simulink model "EV_Truck_Model"  (R2022b)
settings: Solver=FixedStepAuto  StartTime=0  StopTime=26553  FixedStep=0.1  RelTol=1e-3
model workspace (MAT data in the model file):
  ADAS_MaxAccel = 2
  ADAS_MaxDecel = 2.5
  Adas_on_off = 0
  Batt_cap_ah : Simulink.Parameter (value not decoded)
  Batt_rist_r0 : Simulink.Parameter (value not decoded)
  Batt_soc_s0 : Simulink.Parameter (value not decoded)
  Batt_volt_v0 : Simulink.Parameter (value not decoded)
  Motor_eff_100 : Simulink.Parameter (value not decoded)
  Motor_eff_190 : Simulink.Parameter (value not decoded)
  Motor_eff_95 : Simulink.Parameter (value not decoded)
  Motor_rpm_100 : Simulink.Parameter (value not decoded)
  Motor_rpm_190 : Simulink.Parameter (value not decoded)
  Motor_rpm_95 : Simulink.Parameter (value not decoded)
  Motor_torque_pos_100 : Simulink.Parameter (value not decoded)
  Motor_torque_pos_190 : Simulink.Parameter (value not decoded)
  Motor_torque_pos_95 : Simulink.Parameter (value not decoded)
  Motor_trq_190 : Simulink.Parameter (value not decoded)
  Motor_trq_95 : Simulink.Parameter (value not decoded)
  Sim_step = 0.1
  Test_DriveCycle = 0
  Trans_ratio = 6.142
  Veh_cog_fx = 1.69543
  Veh_cog_h = 0.605887
  Veh_cog_rx = 2.11956
  Veh_diff = 6.7
  Veh_whl_crr = 0.01
  Veh_whl_k = 180000
  Veh_whl_radius = 0.35
symbols that are objects in the model workspace (value not decoded): Motor_eff_100, Motor_eff_190, Motor_eff_95, Motor_rpm_100, Motor_rpm_190, Motor_rpm_95, Motor_torque_pos_100, Motor_torque_pos_190, Motor_torque_pos_95, Motor_trq_190, Motor_trq_95
undefined symbols (not defined in the file): Batt_soc_init, canChannel, Elec_aux_sw, Elec_rgn_sw, Power_option, speed, time, Veh_mass
libraries: batteryecm_lib x170, simulink x14, canmsglib x9, canlib x7, autolibshared x5, nesl_utility x4, fl_lib x3, drivingvehiclecontroller x3, hdlsllib x3, sim3dlib x1, sim3dautolib x1, vrlib x1
(part 4 of 11)

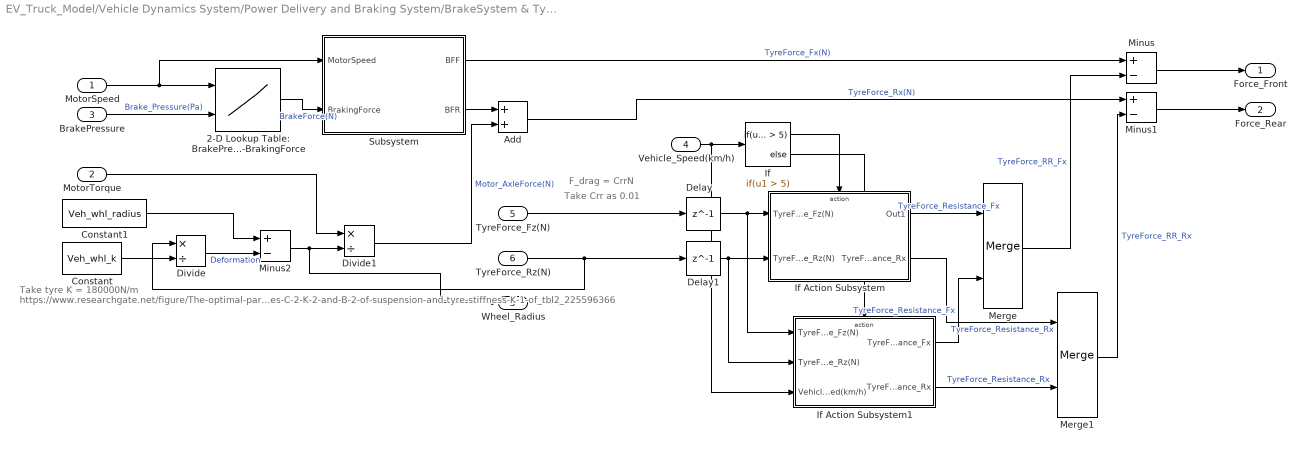
== system EV_Truck_Model/Vehicle Dynamics System/Power Delivery and Braking System/BrakeSystem & Tyre Rolling Resistance ==
  note: Take tyre K = 180000N/m
      | https://www.researchgate.net/figure/The-optimal-parameter-values-C-2-K-2-and-B-2-of-suspension-and-tyre-stiffness-K-1-of_tbl2_225596366
  note: F_drag = CrrN
  note: Take Crr as 0.01
  MotorSpeed : Inport
  MotorTorque : Inport  Port=2
  BrakePressure : Inport  Port=3
  Vehicle_Speed(km/h) : Inport  Port=4
  TyreForce_Fz(N) : Inport  Port=5
  TyreForce_Rz(N) : Inport  Port=6
  2-D Lookup Table: BrakePressure/MotorSpeed-BrakingForce : Lookup_n-D  BreakpointsForDimension1=[0;5000]  BreakpointsForDimension2=[0;1000000000]  Table=[0 32000;0 22800]  InternalRulePriority=Speed  RndMeth=Simplest
      settings: InputPortMap=u0,u1
  Add : Sum
  Constant : Constant  Value=Veh_whl_k
  Constant1 : Constant  Value=Veh_whl_radius
  Delay : Delay  DelayLength=1
  Delay1 : Delay  DelayLength=1
  Divide : Product  Inputs=*/
  Divide1 : Product  Inputs=*/
  If : If  IfExpression=u1 > 5
  If Action Subsystem : Subsystem  TreatAsAtomicUnit=on
  If Action Subsystem1 : Subsystem  TreatAsAtomicUnit=on
  Merge : Merge
  Merge1 : Merge
  Minus : Sum  Inputs=+-
  Minus1 : Sum  Inputs=+-
  Minus2 : Sum  Inputs=+-
  Subsystem : Subsystem
  Force_Front : Outport
  Force_Rear : Outport  Port=2
  Wheel_Radius : Outport  Port=3
  wires:
  TyreForce_Fz(N)/1 -> Delay/1
  TyreForce_Rz(N)/1 -> Divide/1, Delay1/1
  Merge/1 -> Minus/2  "TyreForce_RR_Fx"
  Merge1/1 -> Minus1/2  "TyreForce_RR_Rx"
  Minus1/1 -> Force_Rear/1
  Minus/1 -> Force_Front/1
  Vehicle_Speed(km/h)/1 -> If/1, If Action Subsystem1/3(Vehicle_Speed(km/h))
  If/1 -> If Action Subsystem/Action
  If/2 -> If Action Subsystem1/Action
  If Action Subsystem1/1(TyreForce_Resistance_Fx) -> Merge/2  "TyreForce_Resistance_Fx"
  If Action Subsystem/1(Out1) -> Merge/1  "TyreForce_Resistance_Fx"
  If Action Subsystem1/2(TyreForce_Resistance_Rx) -> Merge1/2  "TyreForce_Resistance_Rx"
  If Action Subsystem/2(TyreForce_Resistance_Rx) -> Merge1/1  "TyreForce_Resistance_Rx"
  Delay/1 -> If Action Subsystem1/1(TyreForce_Fz(N)), If Action Subsystem/1(TyreForce_Fz(N))
  Delay1/1 -> If Action Subsystem1/2(TyreForce_Rz(N)), If Action Subsystem/2(TyreForce_Rz(N))
  Add/1 -> Minus1/1  "TyreForce_Rx(N)"
  Subsystem/1(BFF) -> Minus/1  "TyreForce_Fx(N)"
  MotorSpeed/1 -> Subsystem/1(MotorSpeed), 2-D Lookup Table: BrakePressure/MotorSpeed-BrakingForce/1
  Divide1/1 -> Add/2  "Motor_AxleForce(N)"
  Subsystem/2(BFR) -> Add/1
  2-D Lookup Table: BrakePressure/MotorSpeed-BrakingForce/1 -> Subsystem/2(BrakingForce)  "BrakeForce(N)"
  BrakePressure/1 -> 2-D Lookup Table: BrakePressure/MotorSpeed-BrakingForce/2  "Brake_Pressure(Pa)"
  MotorTorque/1 -> Divide1/1
  Constant/1 -> Divide/2
  Constant1/1 -> Minus2/1
  Divide/1 -> Minus2/2  "Deformation"
  Minus2/1 -> Wheel_Radius/1, Divide1/2

== system EV_Truck_Model/Vehicle Dynamics System/Power Delivery and Braking System/GearBox ==
  AxleTorque : Inport
  Chart : Stateflow chart  Commented=on  TreatAsAtomicUnit=on
  DrivingTorque : Outport
  wires:
  AxleTorque/1 -> DrivingTorque/1
